simulink model "Aircraft6dof_forTrimAndLin_ATT_wInputs1"  (R2023b)
settings: Solver=ode4  StartTime=startTime  StopTime=stopTime  FixedStep=stepTime  RelTol=1e-3  EnableMultiTasking=on
values from neighbouring files (symbols this model uses):
  a0_s2 = 0    [SetupForTrimAndLin_Aircraft6dof.m]
  a0_s3 = 0    [SetupForTrimAndLin_Aircraft6dof.m]
  a0_s4 = 0.05    [SetupForTrimAndLin_Aircraft6dof.m]
  a0_s5 = 0.05    [SetupForTrimAndLin_Aircraft6dof.m]
  AR_s2 = b_s2 / c_s2    [SetupForTrimAndLin_Aircraft6dof.m]
  AR_s3 = b_s3 / c_s3    [SetupForTrimAndLin_Aircraft6dof.m]
  AR_s4 = (b_s4+b_s5) / c_s4    [SetupForTrimAndLin_Aircraft6dof.m]
  AR_s5 = (b_s4+b_s5) / c_s5    [SetupForTrimAndLin_Aircraft6dof.m]
  c_s2 = componentMassesAndGeom(3,2)    [SetupForTrimAndLin_Aircraft6dof.m]
  c_s3 = componentMassesAndGeom(4,2)    [SetupForTrimAndLin_Aircraft6dof.m]
  c_s4 = componentMassesAndGeom(1,2)    [SetupForTrimAndLin_Aircraft6dof.m]
  c_s5 = componentMassesAndGeom(2,2)    [SetupForTrimAndLin_Aircraft6dof.m]
  CD0_s2 = 0.01    [SetupForTrimAndLin_Aircraft6dof.m]
  CD0_s3 = 0.01    [SetupForTrimAndLin_Aircraft6dof.m]
  CD0_s4 = 0.01    [SetupForTrimAndLin_Aircraft6dof.m]
  CD0_s5 = 0.01    [SetupForTrimAndLin_Aircraft6dof.m]
  CDa_s2 = 1    [SetupForTrimAndLin_Aircraft6dof.m]
  CDa_s3 = 1    [SetupForTrimAndLin_Aircraft6dof.m]
  CDa_s4 = 1    [SetupForTrimAndLin_Aircraft6dof.m]
  CDa_s5 = 1    [SetupForTrimAndLin_Aircraft6dof.m]
  CL0_s2 = 0    [SetupForTrimAndLin_Aircraft6dof.m]
  CL0_s3 = 0    [SetupForTrimAndLin_Aircraft6dof.m]
  CL0_s4 = 0.05    [SetupForTrimAndLin_Aircraft6dof.m]
  CL0_s5 = 0.05    [SetupForTrimAndLin_Aircraft6dof.m]
  CM0_s2 = 0    [SetupForTrimAndLin_Aircraft6dof.m]
  CM0_s3 = 0    [SetupForTrimAndLin_Aircraft6dof.m]
  CM0_s4 = -0.05    [SetupForTrimAndLin_Aircraft6dof.m]
  CM0_s5 = -0.05    [SetupForTrimAndLin_Aircraft6dof.m]
  CMa_s2 = 0    [SetupForTrimAndLin_Aircraft6dof.m]
  CMa_s3 = 0    [SetupForTrimAndLin_Aircraft6dof.m]
  CMa_s4 = 0    [SetupForTrimAndLin_Aircraft6dof.m]
  CMa_s5 = 0    [SetupForTrimAndLin_Aircraft6dof.m]
  dCL_du = 3    [SetupForTrimAndLin_Aircraft6dof.m]
  dE_0 = 0    [SetupForTrimAndLin_Aircraft6dof.m]
  dEL_0 = 0    [SetupForTrimAndLin_Aircraft6dof.m]
  dER_0 = 0    [SetupForTrimAndLin_Aircraft6dof.m]
  dR_0 = 0    [SetupForTrimAndLin_Aircraft6dof.m]
  e_s2 = 0.8    [SetupForTrimAndLin_Aircraft6dof.m]
  e_s3 = 0.8    [SetupForTrimAndLin_Aircraft6dof.m]
  e_s4 = 0.9    [SetupForTrimAndLin_Aircraft6dof.m]
  e_s5 = 0.9    [SetupForTrimAndLin_Aircraft6dof.m]
  g_E_N = [0; 0; 9.81]*1    [SetupAndRun_Aircraft6dof.m]    (also in SetupForTrimAndLin_Aircraft6dof.m = [0; 0; 9.81])
  i_s2 = -0.1    [SetupForTrimAndLin_Aircraft6dof.m]
  i_s3 = 0    [SetupForTrimAndLin_Aircraft6dof.m]
  i_s4 = 0.0    (= 0)    [SetupForTrimAndLin_Aircraft6dof.m]
  i_s5 = 0.0    (= 0)    [SetupForTrimAndLin_Aircraft6dof.m]
  InitAtt = InitAtt_deg * deg2rad    [SetupAndRun_Aircraft6dof.m]    (also in SetupForTrimAndLin_Aircraft6dof.m)
  InitPos = InitPos_deg .* [deg2rad; deg2rad; 1]    [SetupAndRun_Aircraft6dof.m]    (also in SetupForTrimAndLin_Aircraft6dof.m)
  InitRates = Rates_Trim    [SetupAndRun_Aircraft6dof.m]    (also in SetupForTrimAndLin_Aircraft6dof.m = [0; 0; 0])
  InitVel = Vel_B_BA_Trim    [SetupAndRun_Aircraft6dof.m]    (also in SetupForTrimAndLin_Aircraft6dof.m = [15; 0; 0])
  J = zeros(3,3)    [DefineAircraftGeometry.m]    (also in InitializeModel.m = ASW.RotationalInertiaMatrix; SetupAndRun_Aircraft6dof.m = [0.049 0 -0.0004; 0 0.022 0; -0.0004 0 0.071]; SetupForTrimAndLin_Aircraft6dof.m)
  m = sum(obj.componentMassesAndGeom(:,1))    [DefineAircraftGeometry.m]    (also in SetupForTrimAndLin_Aircraft6dof.m = sum(componentMassesAndGeom(:,1)))
  MixMatrix = [-1 1 0 0 ... (first row only)    [SetupForTrimAndLin_Aircraft6dof.m]
  n_s2 = [0; 0; -1]    [SetupForTrimAndLin_Aircraft6dof.m]
  n_s3 = [0; 1; 0]    [SetupForTrimAndLin_Aircraft6dof.m]
  n_s4 = [0; sin(0*pi/180);  -cos(0*pi/180)]    [SetupForTrimAndLin_Aircraft6dof.m]
  n_s5 = [0; sin(0*pi/180);  -cos(0*pi/180)]    [SetupForTrimAndLin_Aircraft6dof.m]
  om_motor_init = 0    [SetupForTrimAndLin_Aircraft6dof.m]
  omDot_motor = 0    [SetupForTrimAndLin_Aircraft6dof.m]
  S_s2 = c_s2 * b_s2    [SetupForTrimAndLin_Aircraft6dof.m]
  S_s3 = c_s3 * b_s3    [SetupForTrimAndLin_Aircraft6dof.m]
  S_s4 = c_s4 * b_s4    [SetupForTrimAndLin_Aircraft6dof.m]
  S_s5 = c_s5 * b_s5    [SetupForTrimAndLin_Aircraft6dof.m]
  S_u_s2 = c_u_s2*b_s2    [SetupForTrimAndLin_Aircraft6dof.m]
  S_u_s3 = c_u_s3*b_s3    [SetupForTrimAndLin_Aircraft6dof.m]
  S_u_s4 = c_u_s4*b_s4    [SetupForTrimAndLin_Aircraft6dof.m]
  S_u_s5 = c_u_s5*b_s5    [SetupForTrimAndLin_Aircraft6dof.m]
  tauE = 0.1    [SetupForTrimAndLin_Aircraft6dof.m]
  tauEL = 0.1    [SetupForTrimAndLin_Aircraft6dof.m]
  tauER = 0.1    [SetupForTrimAndLin_Aircraft6dof.m]
  tauR = 0.1    [SetupForTrimAndLin_Aircraft6dof.m]
  v_N_AE = [0; 0; 0]    [SetupAndRun_Aircraft6dof.m]    (also in SetupForTrimAndLin_Aircraft6dof.m)
  x_cm = sum(obj.componentMassesAndGeom(:,1) .* obj.componentMassesAndGeom(:,5:7)) / m    [DefineAircraftGeometry.m]    (also in SetupForTrimAndLin_Aircraft6dof.m = x_cm')
  x_s2 = [componentMassesAndGeom(3,5) + (1/4)*componentMassesAndGeom(3,2); componentMassesAndGeom(3,6);componentMassesAndGeom(3,7)]    [SetupForTrimAndLin_Aircraft6dof.m]
  x_s3 = [componentMassesAndGeom(4,5) + (1/4)*componentMassesAndGeom(4,2); componentMassesAndGeom(4,6);componentMassesAndGeom(4,7)]    [SetupForTrimAndLin_Aircraft6dof.m]
  x_s4 = [componentMassesAndGeom(1,5) + (1/4)*componentMassesAndGeom(1,2); componentMassesAndGeom(1,6);componentMassesAndGeom(1,7)]    [SetupForTrimAndLin_Aircraft6dof.m]
  x_s5 = [componentMassesAndGeom(2,5) + (1/4)*componentMassesAndGeom(2,2); componentMassesAndGeom(2,6);componentMassesAndGeom(2,7)]    [SetupForTrimAndLin_Aircraft6dof.m]
undefined symbols (not defined in the file or in its folder): InitQuat, J_int, n_int
libraries: vrlib x7, simulink x3
(part 2 of 2)

== system Aircraft6dof_forTrimAndLin_ATT_wInputs1/Equations Of Motion State Equations/QUAT2DCM/Subsystem5 ==
  normal(q) : Inport
  Demux : Demux
  Gain : Gain  Gain=2
  Product1 : Product  RndMeth=Zero
  Product2 : Product  RndMeth=Zero
  Sum : Sum  Inputs=|++
  A31 : Outport
  wires:
  Sum/1 -> Gain/1
  Gain/1 -> A31/1
  normal(q)/1 -> Demux/1
  Demux/3 -> Product1/2
  Demux/2 -> Product2/1
  Demux/4 -> Product2/2
  Product2/1 -> Sum/2
  Product1/1 -> Sum/1
  Demux/1 -> Product1/1

== system Aircraft6dof_forTrimAndLin_ATT_wInputs1/Equations Of Motion State Equations/QUAT2DCM/Subsystem6 ==
  normal(q) : Inport
  Demux : Demux
  Gain : Gain  Gain=2
  Product1 : Product  RndMeth=Zero
  Product2 : Product  RndMeth=Zero
  Sum : Sum  Inputs=|-+
  A32 : Outport
  wires:
  normal(q)/1 -> Demux/1
  Gain/1 -> A32/1
  Demux/3 -> Product2/1
  Demux/2 -> Product1/2
  Demux/1 -> Product1/1
  Sum/1 -> Gain/1
  Product1/1 -> Sum/1
  Product2/1 -> Sum/2
  Demux/4 -> Product2/2

== system Aircraft6dof_forTrimAndLin_ATT_wInputs1/Equations Of Motion State Equations/QUAT2DCM/Subsystem7 ==
  normal(q) : Inport
  Demux : Demux
  Product{,1..3} (4 alike) : Product  RndMeth=Zero
  Sum : Sum  Inputs=+-+-
  A22 : Outport
  wires:
  normal(q)/1 -> Demux/1
  Product/1 -> Sum/4
  Product1/1 -> Sum/3
  Product2/1 -> Sum/2
  Product3/1 -> Sum/1
  Demux/1 -> Product3/1, Product3/2
  Demux/2 -> Product2/1, Product2/2
  Demux/3 -> Product1/1, Product1/2
  Demux/4 -> Product/1, Product/2
  Sum/1 -> A22/1

== system Aircraft6dof_forTrimAndLin_ATT_wInputs1/Equations Of Motion State Equations/QUAT2DCM/Subsystem8 ==
  normal(q) : Inport
  Demux : Demux
  Product{,1..3} (4 alike) : Product  RndMeth=Zero
  Sum : Sum  Inputs=+--+
  A33 : Outport
  wires:
  normal(q)/1 -> Demux/1
  Product/1 -> Sum/4
  Product1/1 -> Sum/3
  Product2/1 -> Sum/2
  Product3/1 -> Sum/1
  Demux/1 -> Product3/1, Product3/2
  Demux/2 -> Product2/1, Product2/2
  Demux/3 -> Product1/1, Product1/2
  Demux/4 -> Product/1, Product/2
  Sum/1 -> A33/1

== system Aircraft6dof_forTrimAndLin_ATT_wInputs1/Equations Of Motion State Equations/QUAT2DCM/norm ==
  q : Inport
  Dot Product : DotProduct  OutDataTypeStr=Inherit: Inherit via internal rule
  Math Function : Math  Operator=sqrt  SignedPower=on
  e/|e| : Product  Inputs=*/  InputSameDT=on  RndMeth=Zero  SaturateOnIntegerOverflow=on  OutDataTypeStr=Inherit: Same as first input
  q/|q| : Outport
  wires:
  q/1 -> Dot Product/2, Dot Product/1, e/|e|/1
  Dot Product/1 -> Math Function/1
  Math Function/1 -> e/|e|/2
  e/|e|/1 -> q/|q|/1

== system Aircraft6dof_forTrimAndLin_ATT_wInputs1/Equations Of Motion State Equations/Rot Dyn (Moments)/Integrate ==
  omDot : Inport
  Constant2 : Constant  Value=InitRates
  Demux : Demux  Outputs=3
  Demux1 : Demux  Outputs=3
  Mux : Mux  Inputs=3
  P : Integrator  InitialConditionSource=external
  Q : Integrator  InitialConditionSource=external
  R : Integrator  InitialConditionSource=external
  om : Outport
  wires:
  Demux1/1 -> P/2
  P/1 -> Mux/1
  Demux/3 -> R/1
  Demux1/3 -> R/2
  Demux1/2 -> Q/2
  Q/1 -> Mux/2
  Demux/2 -> Q/1
  Mux/1 -> om/1
  Constant2/1 -> Demux1/1
  omDot/1 -> Demux/1
  Demux/1 -> P/1
  R/1 -> Mux/3

== system Aircraft6dof_forTrimAndLin_ATT_wInputs1/Equations Of Motion State Equations/Rot Dyn (Moments)/Internal Rotational Component 01 ==
  om_B_B_BE : Inport
  om_int_dot : Inport  Port=2
  Constant1 : Constant  Value=J_int(1)
  Constant3 : Constant  Value=n_int(:,1)
  Cross Product2 : vrlib/Utilities/Cross Product
  Integrate : Subsystem
  Product2 : Product  Inputs=3
  hInt : Outport
  hIntDot : Outport  Port=2
  om_motor : Outport  Port=3
  wires:
  Product2/1 -> Integrate/1(hInt_dot), hIntDot/1
  Cross Product2/1 -> hInt/1
  Constant1/1 -> Product2/2, Integrate/2(J)
  Constant3/1 -> Product2/3, Integrate/3(n)
  om_int_dot/1 -> Product2/1
  om_B_B_BE/1 -> Cross Product2/1
  Integrate/1(hInt) -> Cross Product2/2, om_motor/1

== system Aircraft6dof_forTrimAndLin_ATT_wInputs1/Equations Of Motion State Equations/Rot Kin (Orientation) Euler/Integrate ==
  AttDot : Inport
  Constant1 : Constant  Value=InitAtt
  Demux : Demux  Outputs=3
  Demux1 : Demux  Outputs=3
  Mux : Mux  Inputs=3
  Phi : Integrator  InitialConditionSource=external
  Psi : Integrator  InitialConditionSource=external
  Theta : Integrator  InitialConditionSource=external
  Att : Outport  PortDimensions=3
  wires:
  Demux1/1 -> Phi/2
  Phi/1 -> Mux/1
  Demux/3 -> Psi/1
  Demux1/3 -> Psi/2
  Demux1/2 -> Theta/2
  Theta/1 -> Mux/2
  Demux/2 -> Theta/1
  Mux/1 -> Att/1
  Constant1/1 -> Demux1/1
  AttDot/1 -> Demux/1
  Demux/1 -> Phi/1
  Psi/1 -> Mux/3

== system Aircraft6dof_forTrimAndLin_ATT_wInputs1/Equations Of Motion State Equations/Rot Kin (Orientation) Quaternion/QuatMult ==
  q : Inport
  r : Inport  Port=2
  Mux1 : Mux
  q0 : Subsystem
  q1 : Subsystem
  q2 : Subsystem
  q4 : Subsystem
  q*r : Outport
  wires:
  q/1 -> q4/1(q), q2/1(q), q1/1(q), q0/1(q)
  Mux1/1 -> q*r/1
  q0/1(q0) -> Mux1/1
  q4/1(q3) -> Mux1/4
  q1/1(q1) -> Mux1/2
  q2/1(q2) -> Mux1/3
  r/1 -> q4/2(r), q2/2(r), q1/2(r), q0/2(r)

== system Aircraft6dof_forTrimAndLin_ATT_wInputs1/Equations Of Motion State Equations/Rot Kin (Orientation) Quaternion/norm1 ==
  q : Inport
  Dot Product : DotProduct  OutDataTypeStr=Inherit: Inherit via internal rule
  Math Function : Math  Operator=sqrt  SignedPower=on
  e/|e| : Product  Inputs=*/  InputSameDT=on  RndMeth=Zero  SaturateOnIntegerOverflow=on  OutDataTypeStr=Inherit: Same as first input
  q/|q| : Outport
  wires:
  e/|e|/1 -> q/|q|/1
  Math Function/1 -> e/|e|/2
  Dot Product/1 -> Math Function/1
  q/1 -> e/|e|/1, Dot Product/1, Dot Product/2

== system Aircraft6dof_forTrimAndLin_ATT_wInputs1/Equations Of Motion State Equations/Trans Dyn (Forces)/Integrate ==
  VelDot : Inport
  Constant2 : Constant  Value=InitVel
  Demux : Demux  Outputs=3
  Demux1 : Demux  Outputs=3
  Mux : Mux  Inputs=3
  U : Integrator  InitialConditionSource=external
  V : Integrator  InitialConditionSource=external
  W : Integrator  InitialConditionSource=external
  Vel : Outport
  wires:
  Demux1/1 -> U/2
  U/1 -> Mux/1
  Demux/3 -> W/1
  Demux1/3 -> W/2
  Demux1/2 -> V/2
  V/1 -> Mux/2
  Demux/2 -> V/1
  Mux/1 -> Vel/1
  Constant2/1 -> Demux1/1
  VelDot/1 -> Demux/1
  Demux/1 -> U/1
  W/1 -> Mux/3

== system Aircraft6dof_forTrimAndLin_ATT_wInputs1/Equations Of Motion State Equations/Trans Kin (Spherical)/LatDot ==
  Vn : Inport
  Rearth : Inport  Port=2
  alt : Inport  Port=3
  Add : Sum
  Divide : Product  Inputs=*/
  latDot : Outport
  wires:
  Vn/1 -> Divide/1
  Add/1 -> Divide/2
  Divide/1 -> latDot/1
  alt/1 -> Add/2
  Rearth/1 -> Add/1

== system Aircraft6dof_forTrimAndLin_ATT_wInputs1/Equations Of Motion State Equations/Trans Kin (Spherical)/LonDot ==
  Ve : Inport
  Rearth : Inport  Port=2
  alt : Inport  Port=3
  lat : Inport  Port=4
  Add1 : Sum
  Divide1 : Product  Inputs=*//
  Trigonometric Function : Trigonometry  Operator=cos
  lonDot : Outport
  wires:
  Ve/1 -> Divide1/1
  Add1/1 -> Divide1/2
  lat/1 -> Trigonometric Function/1
  Trigonometric Function/1 -> Divide1/3
  Divide1/1 -> lonDot/1
  Rearth/1 -> Add1/1
  alt/1 -> Add1/2

== system Aircraft6dof_forTrimAndLin_ATT_wInputs1/Equations Of Motion State Equations/Trans Kin (Spherical)/wrap lon ==
  lon : Inport
  Add : Sum  Inputs=-+
  Add1 : Sum
  Compare To Constant : simulink/Logic and Bit Operations/Compare To Constant  relop=>  const=pi  OutDataTypeStr=boolean
  Compare To Constant1 : simulink/Logic and Bit Operations/Compare To Constant  relop=<=  const=-pi  OutDataTypeStr=boolean
  Constant : Constant  Value=2*pi
  Switch : Switch  Criteria=u2 > Threshold  SaturateOnIntegerOverflow=off  InputSameDT=off
  Switch1 : Switch  Criteria=u2 > Threshold  SaturateOnIntegerOverflow=off  InputSameDT=off
  -pi < lon <= pi : Outport
  wires:
  lon/1 -> Compare To Constant/1, Add/2, Switch/3
  Add/1 -> Switch/1
  Compare To Constant/1 -> Switch/2
  Compare To Constant1/1 -> Switch1/2
  Switch/1 -> Switch1/3, Add1/2, Compare To Constant1/1
  Switch1/1 -> -pi < lon <= pi/1
  Constant/1 -> Add/1, Add1/1
  Add1/1 -> Switch1/1

== system Aircraft6dof_forTrimAndLin_ATT_wInputs1/Equations Of Motion State Equations/Rot Dyn (Moments)/Internal Rotational Component 01/Integrate ==
  hInt_dot : Inport
  J : Inport  Port=2
  n : Inport  Port=3
  Constant2 : Constant  Value=om_motor_init
  Demux : Demux  Outputs=3
  Demux1 : Demux  Outputs=3
  Mux : Mux  Inputs=3
  Product1 : Product  Inputs=3
  hx : Integrator  InitialConditionSource=external
  hy : Integrator  InitialConditionSource=external
  hz : Integrator  InitialConditionSource=external
  hInt : Outport
  wires:
  Demux1/1 -> hx/2
  hx/1 -> Mux/1
  Demux/3 -> hz/1
  Demux1/3 -> hz/2
  Demux1/2 -> hy/2
  hy/1 -> Mux/2
  Demux/2 -> hy/1
  Mux/1 -> hInt/1
  Product1/1 -> Demux1/1
  hInt_dot/1 -> Demux/1
  Demux/1 -> hx/1
  hz/1 -> Mux/3
  Constant2/1 -> Product1/3
  n/1 -> Product1/2
  J/1 -> Product1/1

== system Aircraft6dof_forTrimAndLin_ATT_wInputs1/Equations Of Motion State Equations/Rot Kin (Orientation) Quaternion/QuatMult/q0 ==
  q : Inport
  r : Inport  Port=2
  Demux : Demux
  Demux1 : Demux
  Product{,1..3} (4 alike) : Product  RndMeth=Zero
  Sum : Sum  Inputs=+---
  q0 : Outport
  wires:
  Product2/1 -> Sum/3
  Sum/1 -> q0/1
  Product3/1 -> Sum/4
  Product1/1 -> Sum/2
  Product/1 -> Sum/1
  Demux/4 -> Product3/1
  Demux1/4 -> Product3/2
  Demux1/3 -> Product2/2
  Demux/3 -> Product2/1
  Demux1/2 -> Product1/2
  Demux/2 -> Product1/1
  Demux1/1 -> Product/2
  Demux/1 -> Product/1
  r/1 -> Demux1/1
  q/1 -> Demux/1

== system Aircraft6dof_forTrimAndLin_ATT_wInputs1/Equations Of Motion State Equations/Rot Kin (Orientation) Quaternion/QuatMult/q1 ==
  q : Inport
  r : Inport  Port=2
  Demux : Demux
  Demux1 : Demux
  Product{,1..3} (4 alike) : Product  RndMeth=Zero
  Sum : Sum  Inputs=+++-
  q1 : Outport
  wires:
  Demux1/3 -> Product3/2
  Demux1/4 -> Product2/2
  Demux1/1 -> Product1/2
  Demux1/2 -> Product/2
  q/1 -> Demux/1
  r/1 -> Demux1/1
  Demux/1 -> Product/1
  Demux/2 -> Product1/1
  Demux/3 -> Product2/1
  Demux/4 -> Product3/1
  Product/1 -> Sum/1
  Product1/1 -> Sum/2
  Product3/1 -> Sum/4
  Sum/1 -> q1/1
  Product2/1 -> Sum/3

== system Aircraft6dof_forTrimAndLin_ATT_wInputs1/Equations Of Motion State Equations/Rot Kin (Orientation) Quaternion/QuatMult/q2 ==
  q : Inport
  r : Inport  Port=2
  Demux : Demux
  Demux1 : Demux
  Product{,1..3} (4 alike) : Product  RndMeth=Zero
  Sum : Sum  Inputs=+-++
  q2 : Outport
  wires:
  Demux1/2 -> Product3/2
  Demux1/1 -> Product2/2
  Demux1/4 -> Product1/2
  Demux1/3 -> Product/2
  Product2/1 -> Sum/3
  Sum/1 -> q2/1
  Product3/1 -> Sum/4
  Product1/1 -> Sum/2
  Product/1 -> Sum/1
  Demux/4 -> Product3/1
  Demux/3 -> Product2/1
  Demux/2 -> Product1/1
  r/1 -> Demux1/1
  q/1 -> Demux/1
  Demux/1 -> Product/1

== system Aircraft6dof_forTrimAndLin_ATT_wInputs1/Equations Of Motion State Equations/Rot Kin (Orientation) Quaternion/QuatMult/q4 ==
  q : Inport
  r : Inport  Port=2
  Demux : Demux
  Demux1 : Demux
  Product{,1..3} (4 alike) : Product  RndMeth=Zero
  Sum : Sum  Inputs=++-+
  q3 : Outport
  wires:
  Demux1/4 -> Product/2
  Demux1/3 -> Product1/2
  Demux1/1 -> Product3/2
  Demux1/2 -> Product2/2
  q/1 -> Demux/1
  r/1 -> Demux1/1
  Demux/1 -> Product/1
  Demux/2 -> Product1/1
  Demux/3 -> Product2/1
  Demux/4 -> Product3/1
  Product/1 -> Sum/1
  Product1/1 -> Sum/2
  Product3/1 -> Sum/4
  Sum/1 -> q3/1
  Product2/1 -> Sum/3

== matlab function Aircraft6dof_forTrimAndLin_ATT_wInputs1/Atmosphere Model/Standard Atmosphere - Troposphere ==
  data: h input; rho output
function rho = fcn(h)
%#codegen

temp_C = 15.04 - 0.00649 * h;
temp_K = 273.15 + temp_C;

press_NQm2 = 101.29 * (temp_K/288.08)^5.256;

rho_kgQm3 = press_NQm2 / (0.2869 *temp_K);

rho = rho_kgQm3;

== matlab function Aircraft6dof_forTrimAndLin_ATT_wInputs1/Equations Of Motion State Equations/Rot Dyn (Moments)/inv of matrix ==
  data: u input; y output
function y = fcn(u)
%#codegen

y = inv(u);

== matlab function Aircraft6dof_forTrimAndLin_ATT_wInputs1/Compute Wind Axes Vector/Compute Wind DCMs ==
  data: Vinf input; C_SB output; C_WB output; alpha input; beta input
function [C_SB, C_WB] = fcn(Vinf, alpha, beta)
%#codegen

C_SB = [cos(alpha)   0   sin(alpha) ;
        0           1   0         ;
        -sin(alpha)  0   cos(alpha)];
    
C_WS = [cos(beta)   sin(beta)   0 ;
        -sin(beta)  cos(beta)   0 ;
        0           0           1];
C_WB = C_WS * C_SB;

== matlab function Aircraft6dof_forTrimAndLin_ATT_wInputs1/Equations Of Motion State Equations/Rot Kin (Orientation) Euler/MATLAB Function ==
  data: ATT input; MATRIX output
function MATRIX = EulerIntegrationMatrix(ATT)
%#codegen

phi=ATT(1);
theta=ATT(2);
psi=ATT(3);

MATRIX = [1     sin(phi)*tan(theta)   cos(phi)*tan(theta) ; 
          0     cos(phi)             -sin(phi)            ;
          0     sin(phi)/cos(theta)   cos(phi)/cos(theta)   ];

== matlab function Aircraft6dof_forTrimAndLin_ATT_wInputs1/Equations Of Motion State Equations/MATLAB Function ==
  data: ATT input; DCM output
function DCM = ATT2DCM(ATT)
%#codegen

phi=ATT(1);
theta=ATT(2);
psi=ATT(3);

DCM = [ cos(theta)*cos(psi)                             cos(theta)*sin(psi)                            -sin(theta)          ; 
        sin(theta)*cos(psi)*sin(phi)-sin(psi)*cos(phi)  sin(theta)*sin(psi)*sin(phi)+cos(psi)*cos(phi)  cos(theta)*sin(phi) ;
        sin(theta)*cos(psi)*cos(phi)+sin(psi)*sin(phi)  sin(theta)*sin(psi)*cos(phi)-cos(psi)*sin(phi)  cos(theta)*cos(phi)   ];
